simulink model "ee_push_pull_converter_ccm"  (R2020a)
settings: Solver=FixedStepAuto  StartTime=0.0  StopTime=0.04  FixedStep=Ts  MaxStep=1e-4  RelTol=1e-3
PreLoadFcn:
  | ee_push_pull_converter_ccm_data;
StopFcn:
  | ee_addSimlogTimeStamp(bdroot)
values from neighbouring files (symbols this model uses):
  Ki = 0.2    [PID_Controller.m]
  Kp = 0.01    [PID_Controller.m]
  Lm = Lr * (m - 1)    [Series_LLC_resonant_converter_calculations.m]    (also in Series_LLC_resonant_converter_calculations_2.m; Series_LLC_resonant_converter_calculations_3.m = Lr / lambda; Transformer_Calculations_Airgap.m = 0.0005265557)
  Rc = lm / (Ur * U0 * Ac)    (= 795774.715459)    [Converter_Magnetics_calculations.m]
undefined symbols (not defined in the file or in its folder): cyclic_load_period, cyclic_load_pul_width, DiscIntNeverNeededParam, fsw_Hz, I_fl_average, Ll, Output_Voltage, primary_winding, R_const, secondary_winding, share_constload, share_cyclicload, Ts
libraries: fl_lib x13, ee_lib x9, nesl_utility x8, simulink x4
CloseFcn:
  | clear simlog_ee_push_pull_converter_ccm
  | clear logsout_ee_push_pull_converter_ccm
Description:
  | Push-Pull Buck Converter in Continuous Conduction Mode
settings Model: Creator=The MathWorks, Inc.  LastModifiedBy=HP
settings SolverCC: AlgebraicLoopSolver=LineSearch
settings DataIOCC: MaxDataPoints=410000  ReturnWorkspaceOutputs=off  SignalLoggingName=logsout_ee_push_pull_converter_ccm
settings OptimizationCC: LifeSpan=inf
settings DebuggingCC: AlgebraicLoopMsg=error  SFExecutionAtInitializationDiag=none  ArithmeticOperatorsInVariantConditions=warning
settings SFSimCC: SimUseLocalCustomCode=off  CustomCodeUndefinedFunction=UseInterfaceOnly
settings RTWCC: RTWUseLocalCustomCode=off
settings CodeAppCC: StateflowObjectComments=on
settings ConfigComp: CovMetricSettings=dswe
settings SimscapeCC: SimscapeLogType=all  SimscapeLogSimulationStatistics=on  SimscapeLogName=simlog_ee_push_pull_converter_ccm  SimscapeLogDataHistory=410000

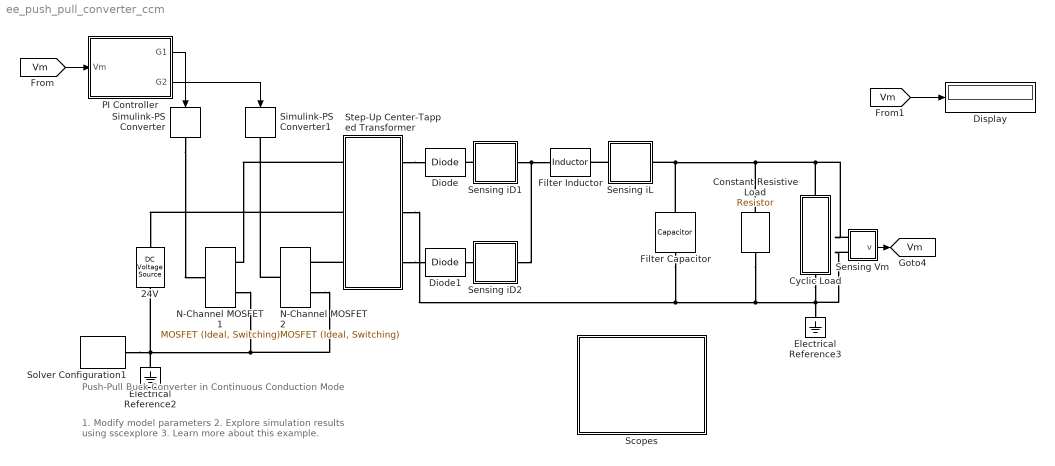
== system ee_push_pull_converter_ccm ==
  note: Push-Pull Buck Converter in Continuous Conduction Mode
  note: 1. Modify model parameters
      | 2. Explore simulation results using sscexplore
      | 3. Learn more about this example.
  " N-Channel MOSFET 1" : ee_lib/Semiconductors & Converters/MOSFET (Ideal, Switching)  Rds=1e-3 Ohm  Goff=1e-6 1/Ohm  Vth=0.5 V  diode_param=1  diode_Vf=0.8 V  diode_Ron=0.001 Ohm  diode_Goff=1e-5 1/Ohm  diode_C=5e-8 F  diode_iRM=-235 A  diode_iF=300 A  diode_idot=-50 A/us  diode_trr_param=1  diode_trr_factor=3  diode_trr=15 us  diode_Qrr=1.5e+3 s*uA  thermal_loss_option=2  Voff=300 V  Tau=1e-4 s  Tj=[298.15, 398.15] K  Iout_scalar=600 A  Eon_scalar=22.86e-3 J  Eoff_scalar=17.14e-3 J  Von_scalar=2.7 V  Iout_data=[0, 10, 50, 100, 200, 400, 600] A  Eon_data=[0, .29, 1.43, 2.86, 5.71, 13.14, 22.86; 0, .57, 2.63, 5.14, 10.29, 20.57, 30.29] * 1e-3 J  Eoff_data=[0, .21, 1.07, 2.14, 4.29, 9.86, 17.14; 0, .43, 1.97, 3.86, 7.71, 15.43, 22.71] * 1e-3 J  Von_data=[0, 1.1, 1.3, 1.45, 1.75, 2.25, 2.7; 0, 1, 1.15, 1.35, 1.7, 2.35, 3] V
  24V : fl_lib/Electrical/Electrical Sources/DC Voltage Source  v0=Input_Voltage V
      settings: SourceProductBaseCode=MT,SS
  Constant Resistive Load : fl_lib/Electrical/Electrical Elements/Resistor  R=R_const/(share_constload*0.01) Ohm  i_specify=off  i_priority=None  i=0 A  i_nominal_specify=off  i_nominal_unit=A  i_nominal_value=1  v_specify=off  v_priority=None  v=0 V  v_nominal_specify=off  v_nominal_unit=V  v_nominal_value=1
      settings: SourceProductBaseCode=MT,SS
  Cyclic Load : Subsystem
  Diode : ee_lib/Semiconductors & Converters/Diode  ModelType=ee.enum.diode.modelType.pwl  Vf=1e-3 V  Ron=0.001 Ohm  Goff=1e-5 1/Ohm  prmExp=ee.enum.diode.expParam.useTwo  I12=[.0137, .545] A  V12=[.6, .7] V  IS=1e-12 A  ec=1  I1=0.0137 A  V1=0.6 V  RS=0 Ohm  Tmeas=25 degC  N_series=1  N_parallel=1  Rz=0.3 Ohm  BV=inf V  C_param=ee.enum.diode.capParam.fixed  CJ=0 pF  CJ0=5 pF  VJ=1 V  Mgrad=0.5  Vvec=[.1, 10, 100] V  Cvec=[3.5, 1, .4] pF  FC=0.5  Q_param=ee.enum.diode.recoveryParam.off  iRM=-7.15 A  iF=4 A  didt=-750 A/us  trr_factor=3  trr=115 ns  Qrr=1500 s*uA  TT=50 ns  tau=100 ns  T_param=ee.enum.diode.temperatureParam.off  IS_T2=1.25e-7 A  I1_T2=0.245 A  V1_T2=0.5 V  Tmeas2=125 degC  EG_param=ee.enum.diode.egapParam.material_si  EG=1.11 eV  XTI_param=ee.enum.diode.xtiParam.pn  XTI=3  dBVdT=0 V/K  Tdevice=25 degC  i_specify=off  i_priority=None  i=0 A  i_nominal_specify=off  i_nominal_unit=A  i_nominal_value=1  v_specify=off  v_priority=None  v=0 V  v_nominal_specify=off  v_nominal_unit=V  v_nominal_value=1  i_capacitor_specify=off  i_capacitor_priority=None  i_capacitor=0 A  i_capacitor_nominal_specify=off  i_capacitor_nominal_unit=A  i_capacitor_nominal_value=1  v_capacitor_specify=off  v_capacitor_priority=None  v_capacitor=0 V  v_capacitor_nominal_specify=off  v_capacitor_nominal_unit=V  v_capacitor_nominal_value=1  power_dissipated_specify=off  power_dissipated_priority=None  power_dissipated=0 W  power_dissipated_nominal_specify=off  power_dissipated_nominal_unit=W  power_dissipated_nominal_value=1  thermal_network_parameterization=ee.enum.thermalNetworkTopology.cauer  Rth=[0, 10] K/W  Rth_Foster=[4, 6] K/W  thermal_mass_parameterization=ee.enum.thermalNetwork.timeconstant  thermal_mass=[0, 1] J/K  thermal_mass_Foster=[1.5, 3] J/K  thermal_time_constant=[0, 10] s  thermal_time_constant_Foster=[6, 18] s  thermal_mass_initial_temperatures=[25, 25] degC
  Diode1 : ee_lib/Semiconductors & Converters/Diode  ModelType=ee.enum.diode.modelType.pwl  Vf=1e-3 V  Ron=0.001 Ohm  Goff=1e-5 1/Ohm  prmExp=ee.enum.diode.expParam.useTwo  I12=[.0137, .545] A  V12=[.6, .7] V  IS=1e-12 A  ec=1  I1=0.0137 A  V1=0.6 V  RS=0 Ohm  Tmeas=25 degC  N_series=1  N_parallel=1  Rz=0.3 Ohm  BV=inf V  C_param=ee.enum.diode.capParam.fixed  CJ=0 pF  CJ0=5 pF  VJ=1 V  Mgrad=0.5  Vvec=[.1, 10, 100] V  Cvec=[3.5, 1, .4] pF  FC=0.5  Q_param=ee.enum.diode.recoveryParam.off  iRM=-7.15 A  iF=4 A  didt=-750 A/us  trr_factor=3  trr=115 ns  Qrr=1500 s*uA  TT=50 ns  tau=100 ns  T_param=ee.enum.diode.temperatureParam.off  IS_T2=1.25e-7 A  I1_T2=0.245 A  V1_T2=0.5 V  Tmeas2=125 degC  EG_param=ee.enum.diode.egapParam.material_si  EG=1.11 eV  XTI_param=ee.enum.diode.xtiParam.pn  XTI=3  dBVdT=0 V/K  Tdevice=25 degC  i_specify=off  i_priority=None  i=0 A  i_nominal_specify=off  i_nominal_unit=A  i_nominal_value=1  v_specify=off  v_priority=None  v=0 V  v_nominal_specify=off  v_nominal_unit=V  v_nominal_value=1  i_capacitor_specify=off  i_capacitor_priority=None  i_capacitor=0 A  i_capacitor_nominal_specify=off  i_capacitor_nominal_unit=A  i_capacitor_nominal_value=1  v_capacitor_specify=off  v_capacitor_priority=None  v_capacitor=0 V  v_capacitor_nominal_specify=off  v_capacitor_nominal_unit=V  v_capacitor_nominal_value=1  power_dissipated_specify=off  power_dissipated_priority=None  power_dissipated=0 W  power_dissipated_nominal_specify=off  power_dissipated_nominal_unit=W  power_dissipated_nominal_value=1  thermal_network_parameterization=ee.enum.thermalNetworkTopology.cauer  Rth=[0, 10] K/W  Rth_Foster=[4, 6] K/W  thermal_mass_parameterization=ee.enum.thermalNetwork.timeconstant  thermal_mass=[0, 1] J/K  thermal_mass_Foster=[1.5, 3] J/K  thermal_time_constant=[0, 10] s  thermal_time_constant_Foster=[6, 18] s  thermal_mass_initial_temperatures=[25, 25] degC
  Display : Display
  Electrical Reference2 : fl_lib/Electrical/Electrical Elements/Electrical Reference
      settings: SourceProductBaseCode=MT,SS
  Electrical Reference3 : fl_lib/Electrical/Electrical Elements/Electrical Reference
      settings: SourceProductBaseCode=MT,SS
  Filter Capacitor : fl_lib/Electrical/Electrical Elements/Capacitor  c=C_min F  r=1e-6 Ohm  g=0 1/Ohm  i_specify=off  i_priority=None  i=0 A  i_nominal_specify=off  i_nominal_unit=A  i_nominal_value=1  v_specify=off  v_priority=None  v=0 V  v_nominal_specify=off  v_nominal_unit=V  v_nominal_value=1  vc_specify=off  vc_priority=High  vc=0 V  vc_nominal_specify=off  vc_nominal_unit=V  vc_nominal_value=1
      settings: SourceProductBaseCode=MT,SS
  Filter Inductor : fl_lib/Electrical/Electrical Elements/Inductor  l=L_min H  r=0 Ohm  g=1e-9 1/Ohm  i_specify=off  i_priority=None  i=0 A  i_nominal_specify=off  i_nominal_unit=A  i_nominal_value=1  v_specify=off  v_priority=None  v=0 V  v_nominal_specify=off  v_nominal_unit=V  v_nominal_value=1  i_L_specify=off  i_L_priority=High  i_L=0 A  i_L_nominal_specify=off  i_L_nominal_unit=A  i_L_nominal_value=1
      settings: SourceProductBaseCode=MT,SS
  N-Channel MOSFET 2 : ee_lib/Semiconductors & Converters/MOSFET (Ideal, Switching)  Rds=1e-3 Ohm  Goff=1e-6 1/Ohm  Vth=0.5 V  diode_param=1  diode_Vf=0.8 V  diode_Ron=0.001 Ohm  diode_Goff=1e-5 1/Ohm  diode_C=5e-8 F  diode_iRM=-235 A  diode_iF=300 A  diode_idot=-50 A/us  diode_trr_param=1  diode_trr_factor=3  diode_trr=15 us  diode_Qrr=1.5e+3 s*uA  thermal_loss_option=2  Voff=300 V  Tau=1e-4 s  Tj=[298.15, 398.15] K  Iout_scalar=600 A  Eon_scalar=22.86e-3 J  Eoff_scalar=17.14e-3 J  Von_scalar=2.7 V  Iout_data=[0, 10, 50, 100, 200, 400, 600] A  Eon_data=[0, .29, 1.43, 2.86, 5.71, 13.14, 22.86; 0, .57, 2.63, 5.14, 10.29, 20.57, 30.29] * 1e-3 J  Eoff_data=[0, .21, 1.07, 2.14, 4.29, 9.86, 17.14; 0, .43, 1.97, 3.86, 7.71, 15.43, 22.71] * 1e-3 J  Von_data=[0, 1.1, 1.3, 1.45, 1.75, 2.25, 2.7; 0, 1, 1.15, 1.35, 1.7, 2.35, 3] V
  PI Controller : Subsystem
  Scopes : Subsystem
  Sensing Vm : Subsystem
  Sensing iD1 : Subsystem
      mask Display: disp('iD1')
  Sensing iD2 : Subsystem
      mask Display: disp('iD2')
  Sensing iL : Subsystem
      mask Display: disp('iL')
  Simulink-PS Converter : nesl_utility/Simulink-PS Converter  PhysicalDomain=network_engine_domain  SubClassName=ps_input  LeftPortType=input  RightPortType=output  PseudoPeriodic=off  Frequencies=[]  NoiseDistribution=none  NoiseParameters=[]  Unit=1  AffineConversion=off  FilteringAndDerivatives=zero  SimscapeFilterOrder=1  InputFilterTimeConstant=0.001  UdotUserProvided=1
      settings: SourceProductBaseCode=MT,SS
  Simulink-PS Converter1 : nesl_utility/Simulink-PS Converter  PhysicalDomain=network_engine_domain  SubClassName=ps_input  LeftPortType=input  RightPortType=output  PseudoPeriodic=off  Frequencies=[]  NoiseDistribution=none  NoiseParameters=[]  Unit=1  AffineConversion=off  FilteringAndDerivatives=zero  SimscapeFilterOrder=1  InputFilterTimeConstant=0.001  UdotUserProvided=1
      settings: SourceProductBaseCode=MT,SS
  Solver Configuration1 : nesl_utility/Solver Configuration  PhysicalDomain=network_engine_domain  SubClassName=solver  LeftPortType=input  RightPortType=generic  Tones=[]  Harmonics=[]  SimulateNoise=off  Profile=off  UseLocalSampling=off  EnableSwitchedLinearOptims=on  FrequencyDomain=off  UseCCode=off  RelTol=0.001  AbsTol=1e-06  MinStep=1e-09  ToWorkspace=off  RevertToSquareIcSolve=off  NumHomotopyIterations=100  PhasorMode=off  PhasorModeNumHarmonics=1  DoDC=off  ResidualTolerance=1e-09  UseLocalSolver=on  LocalSolverChoice=NE_BACKWARD_EULER_ADVANCER  LocalSolverSampleTime=Ts  DoFixedCost=off  MaxNonlinIter=3  MaxModeIter=2  LinearAlgebra=auto  EquationFormulation=NE_TIME_EF  DelaysMemoryBudget=1024  AutomaticFiltering=on  FilteringTimeConstant=0.001  PartitionStorageMethod=AS_NEEDED  PartitionMemoryBudget=1024  PartitionMethod=FAST
      settings: SourceProductBaseCode=MT,SS
  Step-Up Center-Tapped Transformer : Subsystem
  tag scope: Vm=global
  wires:
  Sensing Vm/1(v) -> [Vm]
  PI Controller/2(G2) -> Simulink-PS Converter1/1
  PI Controller/1(G1) -> Simulink-PS Converter/1
  [Vm] -> PI Controller/1(Vm)
  [Vm] -> Display/1
  connections:
  Electrical Reference2/LConn1 -- 24V/RConn1 -- Solver Configuration1/RConn1 -- N-Channel MOSFET 2/RConn2 -- " N-Channel MOSFET 1"/RConn2
  Sensing iD1/RConn1 -- Filter Inductor/LConn1 -- Sensing iD2/RConn1
  Sensing Vm/LConn1 -- Cyclic Load/RConn1 -- Filter Capacitor/LConn1 -- Sensing iL/RConn1 -- Constant Resistive Load/LConn1
  Sensing Vm/LConn2 -- Step-Up Center-Tapped Transformer/RConn2 -- Filter Capacitor/RConn1 -- Constant Resistive Load/RConn1 -- Electrical Reference3/LConn1 -- Cyclic Load/LConn1
  Step-Up Center-Tapped Transformer/LConn2 -- 24V/LConn1
  Step-Up Center-Tapped Transformer/LConn1 -- " N-Channel MOSFET 1"/RConn1
  Step-Up Center-Tapped Transformer/LConn3 -- N-Channel MOSFET 2/RConn1
  Step-Up Center-Tapped Transformer/RConn1 -- Diode/LConn1
  Step-Up Center-Tapped Transformer/RConn3 -- Diode1/LConn1
  Sensing iD1/LConn1 -- Diode/RConn1
  Diode1/RConn1 -- Sensing iD2/LConn1
  Sensing iL/LConn1 -- Filter Inductor/RConn1
  Simulink-PS Converter/RConn1 -- " N-Channel MOSFET 1"/LConn1
  N-Channel MOSFET 2/LConn1 -- Simulink-PS Converter1/RConn1

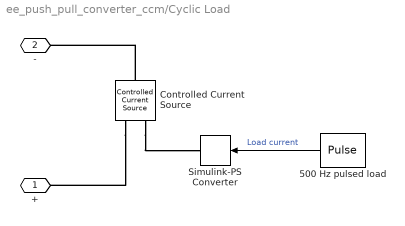
== system ee_push_pull_converter_ccm/Cyclic Load ==
  500 Hz pulsed load : DiscretePulseGenerator  PulseType=Time based  Amplitude=I_fl_average*(share_cyclicload*0.01)  Period=cyclic_load_period  PulseWidth=cyclic_load_pul_width  PhaseDelay=1e-6
  Controlled Current Source : fl_lib/Electrical/Electrical Sources/Controlled Current Source
      settings: SourceProductBaseCode=MT,SS
  Simulink-PS Converter : nesl_utility/Simulink-PS Converter  PhysicalDomain=network_engine_domain  SubClassName=ps_input  LeftPortType=input  RightPortType=output  PseudoPeriodic=off  Frequencies=[]  NoiseDistribution=none  NoiseParameters=[]  Unit=A  AffineConversion=off  FilteringAndDerivatives=zero  SimscapeFilterOrder=1  InputFilterTimeConstant=.001  UdotUserProvided=0
      settings: SourceProductBaseCode=MT,SS
  + : PMIOPort  Side=Right
  - : PMIOPort  Port=2  Side=Left
  wires:
  500 Hz pulsed load/1 -> Simulink-PS Converter/1  "Load current"
  connections:
  Controlled Current Source/RConn2 -- +/RConn1
  Controlled Current Source/LConn1 -- -/RConn1
  Controlled Current Source/RConn1 -- Simulink-PS Converter/RConn1

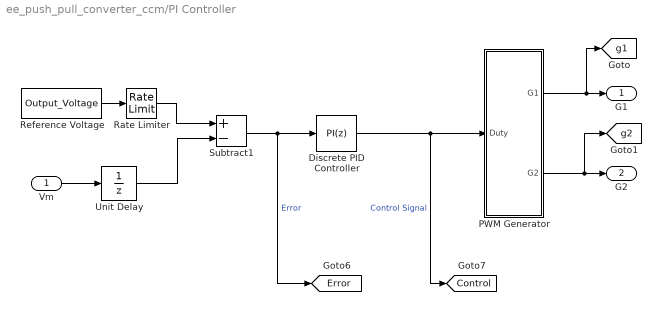
== system ee_push_pull_converter_ccm/PI Controller ==
  Vm : Inport
  Discrete PID Controller : simulink/Continuous/PID Controller  Controller=PI  Form=Parallel  TimeDomain=Discrete-time  UseExternalTs=off  SampleTime=-1  IntegratorMethod=Forward Euler  FilterMethod=Forward Euler  ControllerParametersSource=internal  P=Kp  I=Ki  D=0  UseFilter=on  N=100  TunerSelectOption=Transfer Function Based (PID Tuner App)  InitialConditionSource=internal  InitialConditionForIntegrator=0  InitialConditionForFilter=0  DifferentiatorICPrevScaledInput=0  ExternalReset=none  TrackingMode=off  Kt=1  LimitOutput=on  UpperSaturationLimit=0.5  LowerSaturationLimit=0.01  LinearizeAsGain=off  AntiWindupMode=clamping  Kb=0.1  POutMin=[]  POutMax=[]  IOutMin=[]  IOutMax=[]  DOutMin=[]  DOutMax=[]  NOutMin=[]  NOutMax=[]  SumOutMin=[]  SumOutMax=[]  SaturationOutMin=[]  SaturationOutMax=[]  PParamMin=[]  PParamMax=[]  IParamMin=[]  IParamMax=[]  DParamMin=[]  DParamMax=[]  NParamMin=[]  NParamMax=[]  KbParamMin=[]  KbParamMax=[]  KtParamMin=[]  KtParamMax=[]  KbOutMin=[]  KbOutMax=[]  KtOutMin=[]  KtOutMax=[]  IntegratorOutMin=[]  IntegratorOutMax=[]  FilterOutMin=[]  FilterOutMax=[]  SumI1OutMin=[]  SumI1OutMax=[]  SumI2OutMin=[]  SumI2OutMax=[]  SumI3OutMin=[]  SumI3OutMax=[]  SumI4OutMin=[]  SumI4OutMax=[]  SumDOutMin=[]  SumDOutMax=[]  DifferentiatorOutMin=[]  DifferentiatorOutMax=[]  FilterDiffOutCoefMin=[]  FilterDiffOutCoefMax=[]  ReciprocalOutMin=[]  ReciprocalOutMax=[]  SumDenOutMin=[]  SumDenOutMax=[]  SumNumOutMin=[]  SumNumOutMax=[]  DivideOutMin=[]  DivideOutMax=[]  UdiffTsProdOutMin=[]  UdiffTsProdOutMax=[]  NTsProdOutMin=[]  NTsProdOutMax=[]  UintegralTsProdOutMin=[]  UintegralTsProdOutMax=[]  UngainTsProdOutMin=[]  UngainTsProdOutMax=[]  IntegratorContinuousStateAttributes=''  IntegratorStateMustResolveToSignalObject=off  IntegratorRTWStateStorageClass=Auto  FilterContinuousStateAttributes=''  FilterStateMustResolveToSignalObject=off  FilterRTWStateStorageClass=Auto  ParallelPVariant=InternalParameters  IdealPVariant=Disabled  IVariant=InternalParameters  DVariant=Disabled  IntegratorVariant=Discrete  SatVariant=Enabled  AWVariant=DiscClampingParallel  PCopyVariant=Disabled  TRVariant=Disabled  FdbkBlocksVariant=Forward  IdealPFdbkVariant=Disabled  SatFdbkVariant=Disabled  DerivativeFilterVariant=Disabled  NVariant=Disabled  NCopyVariant=Disabled_SignalSpec  FilterICVariant=Disabled  IntegratorICVariant=InternalICs  ExternalResetVariant=Disabled  TRSumVariant=Passthrough  SumFdbkVariant=Disabled  SumVariant=Sum_PI  TsampFilterVariant=InternalTs  TsampNgainVariant=Passthrough  TsampIntegralVariant=Passthrough
  PWM Generator : Subsystem
  Rate Limiter : RateLimiter  RisingSlewLimit=Output_Voltage/0.01  FallingSlewLimit=-Output_Voltage/0.01  SampleTimeMode=inherited
  Reference Voltage : Constant  Value=Output_Voltage  SampleTime=Ts
  Subtract1 : Sum  Inputs=+-
  Unit Delay : UnitDelay  SampleTime=-1  HasFrameUpgradeWarning=on
  G1 : Outport  VectorParamsAs1DForOutWhenUnconnected=off
  G2 : Outport  Port=2  VectorParamsAs1DForOutWhenUnconnected=off
  tag scope: Control=global, Error=global, g1=global, g2=global
  wires:
  PWM Generator/1(G1) -> [g1], G1/1
  Subtract1/1 -> [Error], Discrete PID Controller/1  "Error"
  Discrete PID Controller/1 -> [Control], PWM Generator/1(Duty)  "Control Signal"
  Vm/1 -> Unit Delay/1
  Unit Delay/1 -> Subtract1/2
  Reference Voltage/1 -> Rate Limiter/1
  PWM Generator/2(G2) -> [g2], G2/1
  Rate Limiter/1 -> Subtract1/1

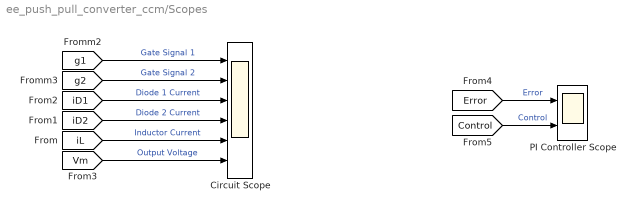
== system ee_push_pull_converter_ccm/Scopes ==
  Circuit Scope : Scope  NumInputPorts=6
  PI Controller Scope : Scope  NumInputPorts=2
  wires:
  [Error] -> PI Controller Scope/1  "Error"
  [iL] -> Circuit Scope/5  "Inductor Current"
  [Vm] -> Circuit Scope/6  "Output Voltage"
  [Control] -> PI Controller Scope/2  "Control"
  [iD2] -> Circuit Scope/4  "Diode 2 Current"
  [iD1] -> Circuit Scope/3  "Diode 1 Current"
  [g1] -> Circuit Scope/1  "Gate Signal 1"
  [g2] -> Circuit Scope/2  "Gate Signal 2"

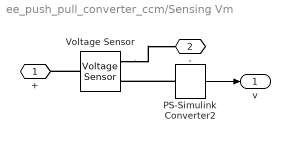
== system ee_push_pull_converter_ccm/Sensing Vm ==
  PS-Simulink Converter2 : nesl_utility/PS-Simulink Converter  PhysicalDomain=network_engine_domain  SubClassName=ps_output  LeftPortType=input  RightPortType=output  PseudoPeriodic=off  Frequencies=[]  Unit=1  AffineConversion=off
      settings: SourceProductBaseCode=MT,SS
  Voltage Sensor : fl_lib/Electrical/Electrical Sensors/Voltage Sensor
      settings: SourceProductBaseCode=MT,SS
  + : PMIOPort  Side=Left
  - : PMIOPort  Port=2  Side=Left
  v : Outport  VectorParamsAs1DForOutWhenUnconnected=off
  wires:
  PS-Simulink Converter2/1 -> v/1
  connections:
  PS-Simulink Converter2/LConn1 -- Voltage Sensor/RConn1
  Voltage Sensor/LConn1 -- +/RConn1
  Voltage Sensor/RConn2 -- -/RConn1

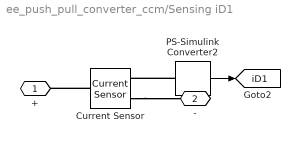
== system ee_push_pull_converter_ccm/Sensing iD1 ==
  Current Sensor : fl_lib/Electrical/Electrical Sensors/Current Sensor
      settings: SourceProductBaseCode=MT,SS
  PS-Simulink Converter2 : nesl_utility/PS-Simulink Converter  PhysicalDomain=network_engine_domain  SubClassName=ps_output  LeftPortType=input  RightPortType=output  PseudoPeriodic=off  Frequencies=[]  Unit=1  AffineConversion=off
      settings: SourceProductBaseCode=MT,SS
  + : PMIOPort  Side=Left
  - : PMIOPort  Port=2  Side=Right
  tag scope: iD1=global
  wires:
  PS-Simulink Converter2/1 -> [iD1]
  connections:
  Current Sensor/LConn1 -- +/RConn1
  Current Sensor/RConn2 -- -/RConn1
  PS-Simulink Converter2/LConn1 -- Current Sensor/RConn1

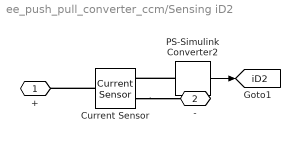
== system ee_push_pull_converter_ccm/Sensing iD2 ==
  Current Sensor : fl_lib/Electrical/Electrical Sensors/Current Sensor
      settings: SourceProductBaseCode=MT,SS
  PS-Simulink Converter2 : nesl_utility/PS-Simulink Converter  PhysicalDomain=network_engine_domain  SubClassName=ps_output  LeftPortType=input  RightPortType=output  PseudoPeriodic=off  Frequencies=[]  Unit=1  AffineConversion=off
      settings: SourceProductBaseCode=MT,SS
  + : PMIOPort  Side=Left
  - : PMIOPort  Port=2  Side=Right
  tag scope: iD2=global
  wires:
  PS-Simulink Converter2/1 -> [iD2]
  connections:
  PS-Simulink Converter2/LConn1 -- Current Sensor/RConn1
  Current Sensor/RConn2 -- -/RConn1
  Current Sensor/LConn1 -- +/RConn1

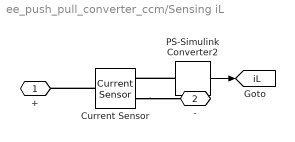
== system ee_push_pull_converter_ccm/Sensing iL ==
  Current Sensor : fl_lib/Electrical/Electrical Sensors/Current Sensor
      settings: SourceProductBaseCode=MT,SS
  PS-Simulink Converter2 : nesl_utility/PS-Simulink Converter  PhysicalDomain=network_engine_domain  SubClassName=ps_output  LeftPortType=input  RightPortType=output  PseudoPeriodic=off  Frequencies=[]  Unit=1  AffineConversion=off
      settings: SourceProductBaseCode=MT,SS
  + : PMIOPort  Side=Left
  - : PMIOPort  Port=2  Side=Right
  tag scope: iL=global
  wires:
  PS-Simulink Converter2/1 -> [iL]
  connections:
  PS-Simulink Converter2/LConn1 -- Current Sensor/RConn1
  Current Sensor/RConn2 -- -/RConn1
  Current Sensor/LConn1 -- +/RConn1

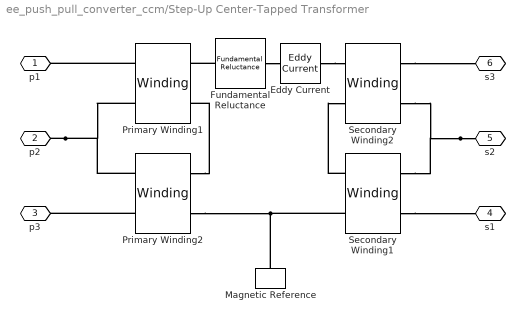
== system ee_push_pull_converter_ccm/Step-Up Center-Tapped Transformer ==
  Eddy Current : ee_lib/Passive/Eddy Current  g=primary_winding^2/Rc 1/Ohm  r=0 1/H  p=0 H  phi_L_specify=off  phi_L_priority=None  phi_L=0 Wb  phi_L_nominal_specify=off  phi_L_nominal_unit=Wb  phi_L_nominal_value=1
      settings: SourceProductBaseCode=PS  InternalSimscapePortConfiguration="{\"Bottom\":[],\"Left\":[{\"id\":\"N\",\"label\":\"N\",\"type\":\"foundation.magnetic.magnetic\"}],\"Right\":[{\"id\":\"S\",\"label\":\"S\",\"type\":\"foundation.magnetic.magnetic\"}],\"Top\":[]}"
  Fundamental Reluctance : fl_lib/Magnetic/Magnetic Elements/Fundamental Reluctance  R=primary_winding^2/Lm 1/H  phi_specify=off  phi_priority=None  phi=0 Wb  phi_nominal_specify=off  phi_nominal_unit=Wb  phi_nominal_value=1  mmf_specify=off  mmf_priority=None  mmf=0 A  mmf_nominal_specify=off  mmf_nominal_unit=A  mmf_nominal_value=1
      settings: SourceProductBaseCode=MT,SS  InternalSimscapePortConfiguration="{\"Bottom\":[],\"Left\":[{\"id\":\"N\",\"label\":\"N\",\"type\":\"foundation.magnetic.magnetic\"}],\"Right\":[{\"id\":\"S\",\"label\":\"S\",\"type\":\"foundation.magnetic.magnetic\"}],\"Top\":[]}"
  Magnetic Reference : fl_lib/Magnetic/Magnetic Elements/Magnetic Reference
      settings: SourceProductBaseCode=MT,SS  InternalSimscapePortConfiguration="{\"Bottom\":[],\"Left\":[{\"id\":\"M\",\"label\":\"\",\"type\":\"foundation.magnetic.magnetic\"}],\"Right\":[],\"Top\":[]}"
  Primary Winding1 : ee_lib/Passive/Winding  Nw=primary_winding  Rw=Rw Ohm  Rl=primary_winding^2/Ll 1/H  i_specify=off  i_priority=None  i=0 A  i_nominal_specify=off  i_nominal_unit=A  i_nominal_value=1  phiorg_specify=off  phiorg_priority=High  phiorg=0 Wb  phiorg_nominal_specify=off  phiorg_nominal_unit=Wb  phiorg_nominal_value=1  phi_specify=off  phi_priority=None  phi=0 Wb  phi_nominal_specify=off  phi_nominal_unit=Wb  phi_nominal_value=1
      settings: SourceProductBaseCode=PS  InternalSimscapePortConfiguration="{\"Bottom\":[],\"Left\":[{\"id\":\"p\",\"label\":\"+\",\"type\":\"foundation.electrical.electrical\"},{\"id\":\"n\",\"label\":\"-\",\"type\":\"foundation.electrical.electrical\"}],\"Right\":[{\"id\":\"N\",\"label\":\"N\",\"type\":\"foundation.magnetic.magnetic\"},{\"id\":\"S\",\"label\":\"S\",\"type\":\"foundation.magnetic.magnetic\"}],\"Top\":[]}"
  Primary Winding2 : ee_lib/Passive/Winding  Nw=primary_winding  Rw=Rw Ohm  Rl=primary_winding^2/Ll 1/H  i_specify=off  i_priority=None  i=0 A  i_nominal_specify=off  i_nominal_unit=A  i_nominal_value=1  phiorg_specify=off  phiorg_priority=High  phiorg=0 Wb  phiorg_nominal_specify=off  phiorg_nominal_unit=Wb  phiorg_nominal_value=1  phi_specify=off  phi_priority=None  phi=0 Wb  phi_nominal_specify=off  phi_nominal_unit=Wb  phi_nominal_value=1
      settings: SourceProductBaseCode=PS  InternalSimscapePortConfiguration="{\"Bottom\":[],\"Left\":[{\"id\":\"p\",\"label\":\"+\",\"type\":\"foundation.electrical.electrical\"},{\"id\":\"n\",\"label\":\"-\",\"type\":\"foundation.electrical.electrical\"}],\"Right\":[{\"id\":\"N\",\"label\":\"N\",\"type\":\"foundation.magnetic.magnetic\"},{\"id\":\"S\",\"label\":\"S\",\"type\":\"foundation.magnetic.magnetic\"}],\"Top\":[]}"
  Secondary Winding1 : ee_lib/Passive/Winding  Nw=secondary_winding  Rw=Rw Ohm  Rl=secondary_winding^2/Ll 1/H  i_specify=off  i_priority=None  i=0 A  i_nominal_specify=off  i_nominal_unit=A  i_nominal_value=1  phiorg_specify=off  phiorg_priority=High  phiorg=0 Wb  phiorg_nominal_specify=off  phiorg_nominal_unit=Wb  phiorg_nominal_value=1  phi_specify=off  phi_priority=None  phi=0 Wb  phi_nominal_specify=off  phi_nominal_unit=Wb  phi_nominal_value=1
      settings: SourceProductBaseCode=PS  InternalSimscapePortConfiguration="{\"Bottom\":[],\"Left\":[{\"id\":\"p\",\"label\":\"+\",\"type\":\"foundation.electrical.electrical\"},{\"id\":\"n\",\"label\":\"-\",\"type\":\"foundation.electrical.electrical\"}],\"Right\":[{\"id\":\"N\",\"label\":\"N\",\"type\":\"foundation.magnetic.magnetic\"},{\"id\":\"S\",\"label\":\"S\",\"type\":\"foundation.magnetic.magnetic\"}],\"Top\":[]}"
  Secondary Winding2 : ee_lib/Passive/Winding  Nw=secondary_winding  Rw=Rw Ohm  Rl=secondary_winding^2/Ll 1/H  i_specify=off  i_priority=None  i=0 A  i_nominal_specify=off  i_nominal_unit=A  i_nominal_value=1  phiorg_specify=off  phiorg_priority=High  phiorg=0 Wb  phiorg_nominal_specify=off  phiorg_nominal_unit=Wb  phiorg_nominal_value=1  phi_specify=off  phi_priority=None  phi=0 Wb  phi_nominal_specify=off  phi_nominal_unit=Wb  phi_nominal_value=1
      settings: SourceProductBaseCode=PS  InternalSimscapePortConfiguration="{\"Bottom\":[],\"Left\":[{\"id\":\"p\",\"label\":\"+\",\"type\":\"foundation.electrical.electrical\"},{\"id\":\"n\",\"label\":\"-\",\"type\":\"foundation.electrical.electrical\"}],\"Right\":[{\"id\":\"N\",\"label\":\"N\",\"type\":\"foundation.magnetic.magnetic\"},{\"id\":\"S\",\"label\":\"S\",\"type\":\"foundation.magnetic.magnetic\"}],\"Top\":[]}"
  p1 : PMIOPort  Side=Left
  p2 : PMIOPort  Port=2  Side=Left
  p3 : PMIOPort  Port=3  Side=Left
  s1 : PMIOPort  Port=4  Side=Right
  s2 : PMIOPort  Port=5  Side=Right
  s3 : PMIOPort  Port=6  Side=Right
  connections:
  Primary Winding2/LConn2 -- p3/RConn1
  Primary Winding1/LConn1 -- p1/RConn1
  s2/RConn1 -- Secondary Winding1/LConn2 -- Secondary Winding2/LConn1
  p2/RConn1 -- Primary Winding2/LConn1 -- Primary Winding1/LConn2
  Magnetic Reference/LConn1 -- Secondary Winding1/RConn1 -- Primary Winding2/RConn2
  Primary Winding2/RConn1 -- Primary Winding1/RConn2
  Secondary Winding1/RConn2 -- Secondary Winding2/RConn1
  Secondary Winding1/LConn1 -- s1/RConn1
  Secondary Winding2/LConn2 -- s3/RConn1
  Fundamental Reluctance/RConn1 -- Eddy Current/LConn1
  Eddy Current/RConn1 -- Secondary Winding2/RConn2
  Fundamental Reluctance/LConn1 -- Primary Winding1/RConn1

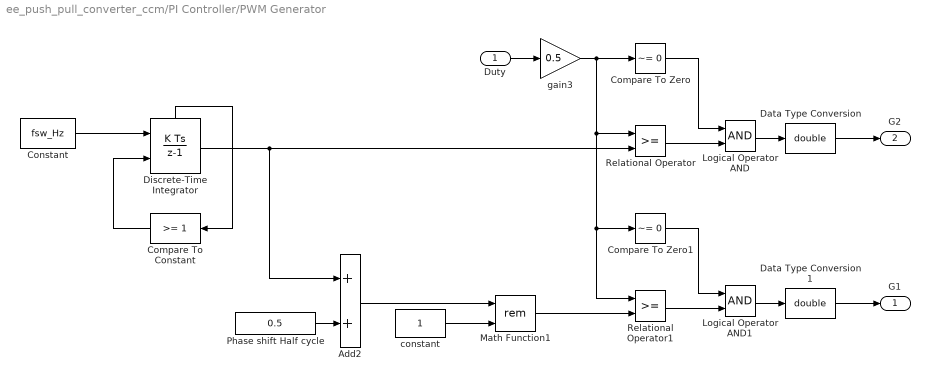
== system ee_push_pull_converter_ccm/PI Controller/PWM Generator ==
  Duty : Inport
  Add2 : Sum
  Compare To Constant : simulink/Logic and Bit Operations/Compare To Constant  relop=>=  const=1  OutDataTypeStr=boolean
  Compare To Zero : simulink/Logic and Bit Operations/Compare To Zero  relop=~=  OutDataTypeStr=boolean
  Compare To Zero1 : simulink/Logic and Bit Operations/Compare To Zero  relop=~=  OutDataTypeStr=boolean
  Constant : Constant  Value=fsw_Hz  SampleTime=Ts
  Data Type Conversion : DataTypeConversion  OutDataTypeStr=double
  Data Type Conversion1 : DataTypeConversion  OutDataTypeStr=double
  Discrete-Time Integrator : DiscreteIntegrator  ExternalReset=rising  SampleTime=-1  ShowStatePort=on  ICPrevOutput=DiscIntNeverNeededParam  ICPrevScaledInput=DiscIntNeverNeededParam
  Logical Operator AND : Logic  AllPortsSameDT=off  OutDataTypeStr=boolean
  Logical Operator AND1 : Logic  AllPortsSameDT=off  OutDataTypeStr=boolean
  Math Function1 : Math  Operator=rem  SignedPower=on  SaturateOnIntegerOverflow=on
  Phase shift Half cycle : Constant  Value=0.5  SampleTime=Ts
  Relational Operator : RelationalOperator  OutDataTypeStr=boolean  RndMeth=Nearest
  Relational Operator1 : RelationalOperator  OutDataTypeStr=boolean  RndMeth=Nearest
  constant : Constant  SampleTime=Ts
  gain3 : Gain  Gain=0.5  SaturateOnIntegerOverflow=on  OutDataTypeStr=Inherit: Same as input  ParamDataTypeStr=Inherit: Same as input
  G1 : Outport  VectorParamsAs1DForOutWhenUnconnected=off
  G2 : Outport  Port=2  VectorParamsAs1DForOutWhenUnconnected=off
  wires:
  Duty/1 -> gain3/1
  Compare To Zero1/1 -> Logical Operator AND1/1
  Compare To Zero/1 -> Logical Operator AND/1
  Relational Operator1/1 -> Logical Operator AND1/2
  Relational Operator/1 -> Logical Operator AND/2
  Phase shift Half cycle/1 -> Add2/2
  Data Type Conversion/1 -> G2/1
  Data Type Conversion1/1 -> G1/1
  Logical Operator AND1/1 -> Data Type Conversion1/1
  Add2/1 -> Math Function1/1
  Math Function1/1 -> Relational Operator1/2
  Logical Operator AND/1 -> Data Type Conversion/1
  constant/1 -> Math Function1/2
  Discrete-Time Integrator/1 -> Relational Operator/2, Add2/1
  gain3/1 -> Compare To Zero/1, Relational Operator/1, Compare To Zero1/1, Relational Operator1/1
  Constant/1 -> Discrete-Time Integrator/1
  Compare To Constant/1 -> Discrete-Time Integrator/2
  Discrete-Time Integrator/State -> Compare To Constant/1
